simulink model "arduino_CAN_simple_example"  (R2014b)
settings: Solver=FixedStepDiscrete  StartTime=0.0  StopTime=10.0  FixedStep=0.1  RelTol=1e-3
libraries: arduino_CAN_library x7, simulink x3, arduinolib x2
settings Model: CovMetricSettings=dwe  CovHtmlReporting=off  covSaveCumulativeToWorkspaceVar=off  CovSaveSingleToWorkspaceVar=off  CovExternalEMLEnable=on  CovSFcnEnable=on  ExtModeTrigDuration=2  Creator=ll2  LastModifiedBy=ll2
settings DataIOCC: LimitDataPoints=off  SaveFormat=StructureWithTime
settings OptimizationCC: PassReuseOutputArgsAs=Individual arguments  OptimizeModelRefInitCode=on  MaxStackSize=64
settings DebuggingCC: SolverPrmCheckMsg=none  ParameterTunabilityLossMsg=error  FrameProcessingCompatibilityMsg=error  SFUnexpectedBacktrackingDiag=error  SFNoUnconditionalDefaultTransitionDiag=error
settings HardwareCC: ProdBitPerInt=16  ProdBitPerPointer=16  ProdIntDivRoundTo=Zero  ProdEndianess=LittleEndian  ProdWordSize=8  ProdHWDeviceType=Atmel->AVR
settings ModelReferenceCC: PropagateSignalLabelsOutOfModel=on
settings RTWCC: SystemTargetFile=ert.tlc  TLCOptions=-aInlineSetEventsForThisBaseRateFcn=TLC_FALSE -aSuppressMultiTaskScheduler=TLC_FALSE -aRateBasedStepFcn=1  TemplateMakefile=ert_default_tmf  Description=Embedded Coder  GenerateReport=on  RTWVerbose=off  CustomInclude="\"..\\..\\externals\\CAN-Bus_Shield\\Libraries\\Canbus\""  CustomSource="\"..\\..\\externals\\CAN-Bus_Shield\\Libraries\\Canbus\\mcp2515.c\""  Toolchain=Arduino AVR  BuildConfiguration=Faster Runs  IncludeHyperlinkInReport=on  LaunchReport=on  GenerateTraceInfo=on  GenerateTraceReport=on  GenerateTraceReportSl=on  GenerateTraceReportSf=on  GenerateTraceReportEml=on
settings CodeAppCC: ForceParamTrailComments=on  IgnoreCustomStorageClasses=off  OperatorAnnotations=on  SimulinkDataObjDesc=on  SFDataObjDesc=on  InsertBlockDesc=on
settings ERTTargetCC: MultiwordLength=256  SupportContinuousTime=on  SupportVariableSizeSignals=on  ConvertIfToSwitch=on  SuppressUnreachableDefaultCases=on

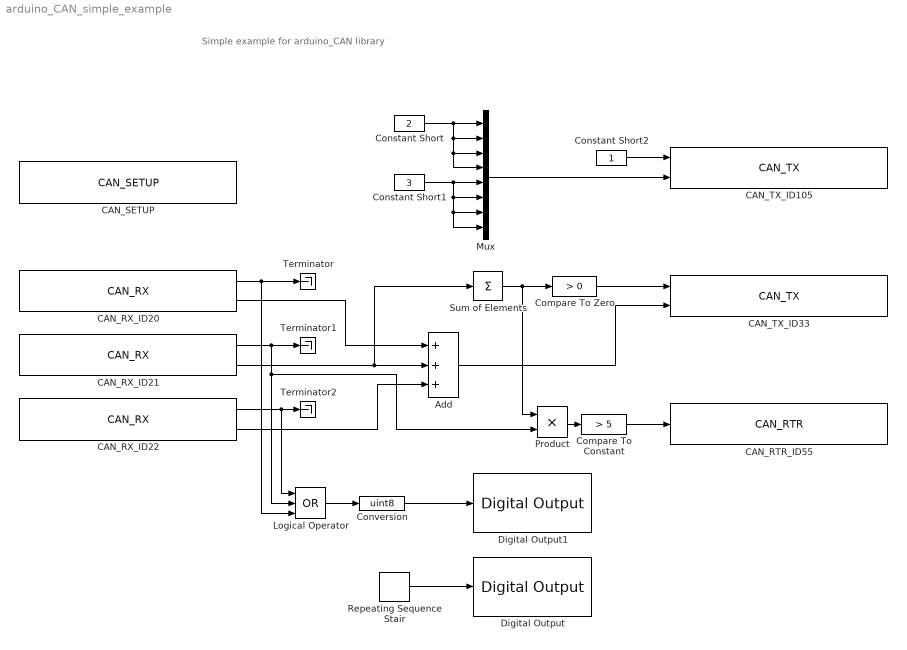
== system arduino_CAN_simple_example ==
  note: Simple example for arduino_CAN library
  Add : Sum  Inputs=+++
  CAN_RTR_ID55 : arduino_CAN_library/CAN_RTR  CANM_ID=55
  CAN_RX_ID20 : arduino_CAN_library/CAN_RX  CANM_ID=20
  CAN_RX_ID21 : arduino_CAN_library/CAN_RX  CANM_ID=21
  CAN_RX_ID22 : arduino_CAN_library/CAN_RX  CANM_ID=22
  CAN_SETUP : arduino_CAN_library/CAN_SETUP  CANIDX=250
  CAN_TX_ID105 : arduino_CAN_library/CAN_TX  CANM_ID=105
  CAN_TX_ID33 : arduino_CAN_library/CAN_TX  CANM_ID=33
  Compare To Constant : simulink/Logic and Bit Operations/Compare To Constant  relop=>  const=5  OutDataTypeStr=uint8  ZeroCross=off
  Compare To Zero : simulink/Logic and Bit Operations/Compare To Zero  relop=>  OutDataTypeStr=uint8  ZeroCross=off
  Constant Short : Constant  Value=2  OutDataTypeStr=uint8
  Constant Short1 : Constant  Value=3  OutDataTypeStr=uint8
  Constant Short2 : Constant  OutDataTypeStr=uint8
  Conversion : DataTypeConversion  OutDataTypeStr=uint8
  Digital Output : arduinolib/Digital Output  pinNumber=7  blockPlatform=arduino
  Digital Output1 : arduinolib/Digital Output  pinNumber=8  blockPlatform=arduino
  Logical Operator : Logic  Operator=OR  Inputs=3  AllPortsSameDT=off  OutDataTypeStr=boolean
  Mux : Mux  Inputs=8
  Product : Product  RndMeth=Zero
  Repeating Sequence Stair : simulink/Sources/Repeating Sequence Stair  OutValues=[1 1 0 1 0 0 1].'  tsamp=0.1  OutMin=[]  OutMax=[]  OutDataTypeStr=uint8  OutputDataTypeScalingMode=uint8  OutDataType=double  ConRadixGroup=Best Precision: Vector-wise  OutScaling=2^-12
  Sum of Elements : Sum  Inputs=+
  Terminator : Terminator
  Terminator1 : Terminator
  Terminator2 : Terminator
  wires:
  Constant Short/1 -> Mux/1, Mux/2, Mux/3, Mux/4
  CAN_RX_ID21/1 -> Terminator1/1, Logical Operator/2, Product/2
  CAN_RX_ID21/2 -> Add/2, Sum of Elements/1
  Add/1 -> CAN_TX_ID33/2
  Compare To Zero/1 -> CAN_TX_ID33/1
  Compare To Constant/1 -> CAN_RTR_ID55/1
  Conversion/1 -> Digital Output1/1
  CAN_RX_ID20/1 -> Terminator/1, Logical Operator/3
  Constant Short2/1 -> CAN_TX_ID105/1
  CAN_RX_ID22/1 -> Terminator2/1, Logical Operator/1
  Mux/1 -> CAN_TX_ID105/2
  Sum of Elements/1 -> Product/1, Compare To Zero/1
  Repeating Sequence Stair/1 -> Digital Output/1
  Logical Operator/1 -> Conversion/1
  Product/1 -> Compare To Constant/1
  CAN_RX_ID20/2 -> Add/1
  Constant Short1/1 -> Mux/5, Mux/6, Mux/7, Mux/8
  CAN_RX_ID22/2 -> Add/3
